simulink model "Commande_floue"  (R2016a)
settings: Solver=VariableStepAuto  StartTime=0.0  StopTime=40  RelTol=1e-3
undefined symbols (not defined in the file): A, Eg, Iscn, K, Ki, Q, Rp, Rse, T, Vocn
libraries: powerlib x14, fuzblock x1, powerlib_extras x1, simulink x1
settings Model: Creator=AIMS  LastModifiedBy=AIMS

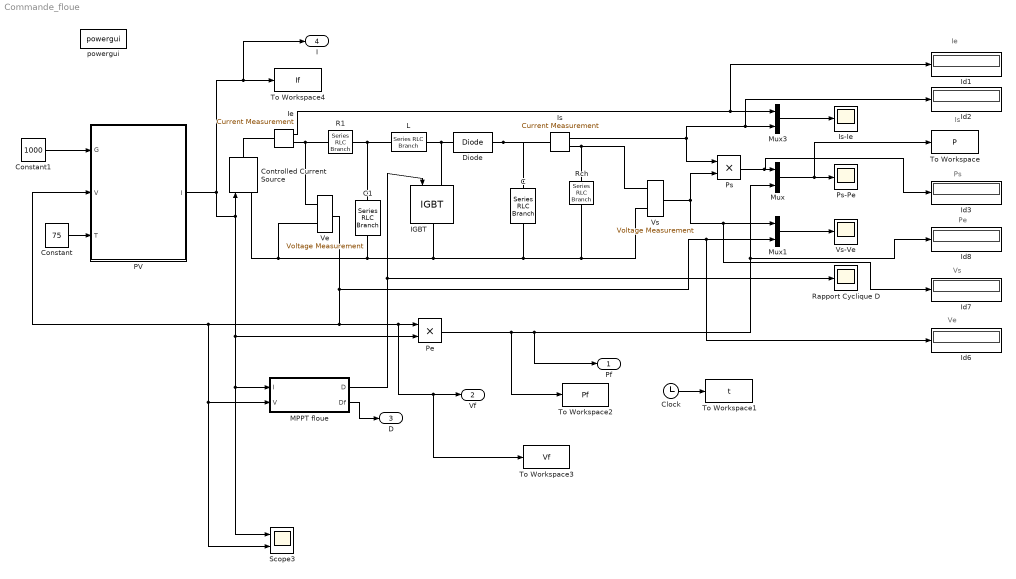
== system Commande_floue ==
  note: Ve
  note: Vs
  note: Pe
  note: Ps
  note: Is
  note: Ie
  C : powerlib/Elements/Series RLC Branch  LConnTagsString=__new0  RConnTagsString=__new0  BranchType=C  Resistance=0.01  Inductance=1.0  SetiL0=off  InitialCurrent=0  Capacitance=400e-6  Setx0=off  InitialVoltage=200  Measurements=None
  C1 : powerlib/Elements/Series RLC Branch  LConnTagsString=__new0  RConnTagsString=__new0  BranchType=C  Resistance=0.01  Inductance=1.0  SetiL0=off  InitialCurrent=0  Capacitance=2e-3  Setx0=off  InitialVoltage=0  Measurements=None
  Clock : Clock
  Constant : Constant  Value=75
  Constant1 : Constant  Value=1000
  Controlled Current Source : powerlib/Electrical Sources/Controlled Current Source  Initialize=on  Source_Type=AC  Amplitude=0  Phase=0  Frequency=0  Measurements=None
  Diode : powerlib/Power Electronics/Diode  Ron=0.001  Lon=0  Vf=0.8  IC=0  UseSnubber=off  Rs=500  Cs=250e-9  Measurements=off
  IGBT : powerlib/Power Electronics/IGBT  Ron=0.001  Lon=0  Vf=1  Tf=1e-6  Tt=2e-6  IC=0  Rs=1e5  Cs=inf  Measurements=off
  Id{1..3,6..8} (6 alike) : Display
  Ie : powerlib/Measurements/Current Measurement  Tag=PoWeRsYsTeMmEaSuReMeNt  PhasorSimulation=off  OutputType=Magnitude  PSBequivalent=0
  Is : powerlib/Measurements/Current Measurement  Tag=PoWeRsYsTeMmEaSuReMeNt  PhasorSimulation=off  OutputType=Magnitude  PSBequivalent=0
  Is-Ie : Scope
  L : powerlib/Elements/Series RLC Branch  LConnTagsString=__new0  RConnTagsString=__new0  BranchType=L  Resistance=1.0  Inductance=76.8e-6  SetiL0=off  InitialCurrent=0  Capacitance=1.0  Setx0=off  InitialVoltage=0  Measurements=None
  MPPT floue : Subsystem
  Mux : Mux  Inputs=2
  Mux1 : Mux  Inputs=2
  Mux3 : Mux  Inputs=2
  PV : Subsystem
  Pe : Product  RndMeth=Zero
  Ps : Product  RndMeth=Zero
  Ps-Pe : Scope
  R1 : powerlib/Elements/Series RLC Branch  LConnTagsString=__new0  RConnTagsString=__new0  BranchType=R  Resistance=0.01  Inductance=1.0  SetiL0=off  InitialCurrent=0  Capacitance=1.0  Setx0=off  InitialVoltage=0  Measurements=None
  Rapport Cyclique D : Scope
  Rch : powerlib/Elements/Series RLC Branch  LConnTagsString=__new0  RConnTagsString=__new0  BranchType=R  Resistance=5  Inductance=1.0  SetiL0=off  InitialCurrent=0  Capacitance=1.0  Setx0=off  InitialVoltage=0  Measurements=None
  Scope3 : Scope  NumInputPorts=2
  To Workspace : ToWorkspace  VariableName=P  SampleTime=-1
  To Workspace1 : ToWorkspace  VariableName=t  SampleTime=-1
  To Workspace2 : ToWorkspace  VariableName=Pf  SampleTime=-1
  To Workspace3 : ToWorkspace  VariableName=Vf  SampleTime=-1
  To Workspace4 : ToWorkspace  VariableName=If  SampleTime=-1
  Ve : powerlib/Measurements/Voltage Measurement  Tag=PoWeRsYsTeMmEaSuReMeNt  PhasorSimulation=off  OutputType=Magnitude  PSBequivalent=0
  Vs : powerlib/Measurements/Voltage Measurement  Tag=PoWeRsYsTeMmEaSuReMeNt  PhasorSimulation=off  OutputType=Magnitude  PSBequivalent=0
  Vs-Ve : Scope
  powergui : powerlib/powergui  SimulationMode=Continuous  SolverType=Tustin  SampleTime=50e-6  frequency=60  SPID=off  DisableSnubberDevices=off  DisableRonSwitches=off  DisableVfSwitches=off  SwTol=0  DisplayEquations=off  Interpol=off  ExternalGateDelay=off  methode=off  Ts=0  FunctionMessages=off  echomessages=off  HookPort=off  EnableUseOfTLC=off  x0status=blocks  frequencyindice=0  Pbase=100e6  ErrMax=1e-4  Iterations=50  UnitsV=kV  UnitsW=MW  buscounter=0  RestoreLinks=warning  ResistiveCurrentMeasurement=off  Frange=[0:2:500]  Ylog=off  Xlog=on  ShowGrid=off  save=off  variable=ZData  structure=mmmm  ZoomFFT=off  StartTime=0.0  cycles=1  DisplayStyle=1  fundamental=60  FreqAxis=off  MaxFrequency=1000  frequencyindicesteady=1  RmsSteady=1  display=off
  Pf : Outport
  Vf : Outport  Port=2
  D : Outport  Port=3
  "I  " : Outport  Port=4
  wires:
  Is/1 -> Id2/1, Mux3/2, Ps/1
  Vs/1 -> Id7/1, Mux1/1, Ps/2
  Pe/1 -> Id8/1, Mux/2, Pf/1, To Workspace2/1
  Ve/1 -> Id6/1, Mux1/2, PV/2(V), Scope3/2, MPPT floue/2(V), Pe/1, Vf/1, To Workspace3/1
  Mux/1 -> Ps-Pe/1, To Workspace/1
  Mux1/1 -> Vs-Ve/1
  Ie/1 -> Id1/1, Mux3/1
  Mux3/1 -> Is-Ie/1
  MPPT floue/1(D) -> Rapport Cyclique D/1, IGBT/1
  Clock/1 -> To Workspace1/1
  MPPT floue/2(Df) -> D/1
  Constant/1 -> PV/3(T)
  PV/1("I ") -> To Workspace4/1, "I  "/1, Controlled Current Source/1, Pe/2, Scope3/1, MPPT floue/1(I)
  Ps/1 -> Id3/1, Mux/1
  Constant1/1 -> PV/1("G ")
  connections:
  Vs/LConn2 -- Rch/RConn1 -- Controlled Current Source/LConn1 -- Ve/LConn2 -- C1/RConn1 -- IGBT/RConn1 -- C/RConn1
  Diode/RConn1 -- C/LConn1 -- Is/LConn1
  Diode/LConn1 -- IGBT/LConn1 -- L/RConn1
  Is/RConn1 -- Vs/LConn1 -- Rch/LConn1
  Ve/LConn1 -- Ie/RConn1 -- R1/RConn1
  R1/LConn1 -- C1/LConn1 -- L/LConn1
  Controlled Current Source/RConn1 -- Ie/LConn1

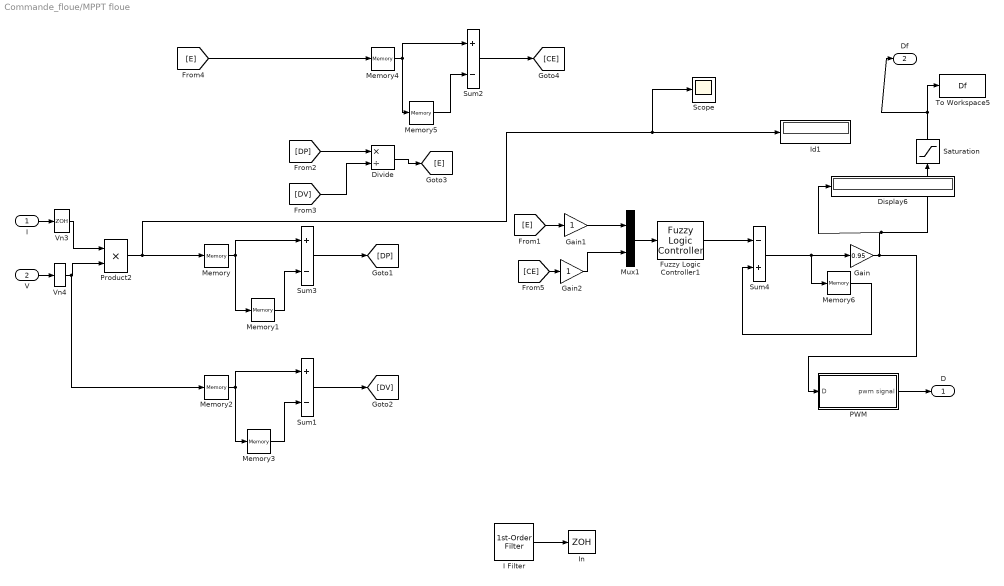
== system Commande_floue/MPPT floue ==
  I : Inport
  V : Inport  Port=2
  Display6 : Display
  Divide : Product  Inputs=*/
  Fuzzy Logic Controller1 : fuzblock/Fuzzy Logic  Controller  fis=sari
  Gain : Gain  Gain=0.95
  Gain1 : Gain
  Gain2 : Gain
  I Filter : powerlib_extras/Control  Blocks/1st-Order  Filter  FilterType=Lowpass  Tc=1e-3  Initialize=off  Vac_Init=[0.8 -25 60]  Vdc_Init=-0.4  PlotResponse=off  param1=[1 500 1]
  Id1 : Display
  In : ZeroOrderHold  SampleTime=4e-4
  Memory{,1..6} (7 alike) : Memory
  Mux1 : Mux  Inputs=2
  PWM : Subsystem
  Product2 : Product
  Saturation : Saturate  UpperLimit=1  LowerLimit=0
  Scope : Scope
  Sum1 : Sum  Inputs=|+-
  Sum2 : Sum  Inputs=|+-
  Sum3 : Sum  Inputs=|+-
  Sum4 : Sum  Inputs=-+
  To Workspace5 : ToWorkspace  VariableName=Df  SampleTime=-1
  Vn3 : ZeroOrderHold  SampleTime=0.01/2
  Vn4 : ZeroOrderHold  SampleTime=0.01/2
  D : Outport
  Df : Outport  Port=2
  wires:
  I/1 -> Vn3/1
  Product2/1 -> Scope/1, Id1/1, Memory/1
  Memory/1 -> Memory1/1, Sum3/1
  Memory1/1 -> Sum3/2
  Sum3/1 -> [DP]
  V/1 -> Vn4/1
  Memory2/1 -> Sum1/1, Memory3/1
  Memory3/1 -> Sum1/2
  Sum1/1 -> [DV]
  [DV] -> Divide/2
  [DP] -> Divide/1
  Divide/1 -> [E]
  [E] -> Memory4/1
  Memory4/1 -> Memory5/1, Sum2/1
  Memory5/1 -> Sum2/2
  Sum2/1 -> [CE]
  Mux1/1 -> Fuzzy Logic Controller1/1
  [E] -> Gain1/1
  [CE] -> Gain2/1
  Fuzzy Logic Controller1/1 -> Sum4/1
  Memory6/1 -> Sum4/2
  Sum4/1 -> Memory6/1, Gain/1
  Gain/1 -> PWM/1(D), Display6/1, Saturation/1
  Gain1/1 -> Mux1/1
  Gain2/1 -> Mux1/2
  ? -> I Filter/1
  I Filter/1 -> In/1
  PWM/1(pwm signal) -> D/1
  Vn3/1 -> Product2/1
  Vn4/1 -> Product2/2, Memory2/1
  Saturation/1 -> To Workspace5/1, Df/1

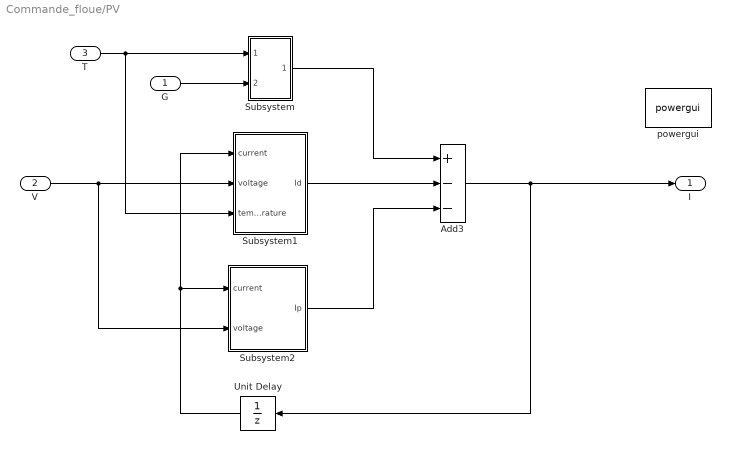
== system Commande_floue/PV ==
  "G " : Inport
  V : Inport  Port=2
  T : Inport  Port=3
  Add3 : Sum  Inputs=+--
  Subsystem : Subsystem
  Subsystem1 : Subsystem
  Subsystem2 : Subsystem
  Unit Delay : UnitDelay
  powergui : powerlib/powergui  Priority=1  SimulationMode=Continuous  SolverType=Tustin/Backward Euler (TBE)  SampleTime=50e-6  frequency=60  SPID=off  DisableSnubberDevices=off  DisableRonSwitches=off  DisableVfSwitches=off  SwTol=0  DisplayEquations=off  Interpol=off  ExternalGateDelay=off  methode=off  Ts=10  FunctionMessages=off  echomessages=off  HookPort=off  EnableUseOfTLC=off  x0status=blocks  frequencyindice=0  Pbase=100e6  ErrMax=1e-4  Iterations=50  UnitsV=kV  UnitsW=MW  buscounter=0  RestoreLinks=warning  ResistiveCurrentMeasurement=off  Frange=[0:2:500]  Ylog=off  Xlog=on  ShowGrid=off  save=off  variable=ZData  structure=0  ZoomFFT=off  StartTime=0.0  cycles=1  DisplayStyle=1  fundamental=60  FreqAxis=off  MaxFrequency=1000  frequencyindicesteady=1  RmsSteady=1  display=off
  "I " : Outport
  wires:
  Add3/1 -> "I "/1, Unit Delay/1
  "G "/1 -> Subsystem/2(In2)
  Unit Delay/1 -> Subsystem2/1("current "), Subsystem1/1(current)
  V/1 -> Subsystem2/2(voltage), Subsystem1/2(voltage)
  Subsystem1/1(Id) -> Add3/2
  Subsystem2/1(Ip) -> Add3/3
  T/1 -> Subsystem1/3(temperature), Subsystem/1(In1)
  Subsystem/1(Iph_out) -> Add3/1

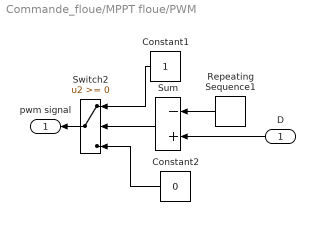
== system Commande_floue/MPPT floue/PWM ==
  D : Inport
  Constant1 : Constant  SampleTime=-1
  Constant2 : Constant  Value=0  SampleTime=-1
  Repeating Sequence1 : simulink/Sources/Repeating Sequence  rep_seq_t=[0 4e-3 4e-2]  rep_seq_y=[0 1 0]
  Sum : Sum  Inputs=-+  SaturateOnIntegerOverflow=on
  Switch2 : Switch
  pwm signal : Outport
  wires:
  Switch2/1 -> pwm signal/1
  Repeating Sequence1/1 -> Sum/1
  Sum/1 -> Switch2/2
  Constant1/1 -> Switch2/1
  Constant2/1 -> Switch2/3
  D/1 -> Sum/2

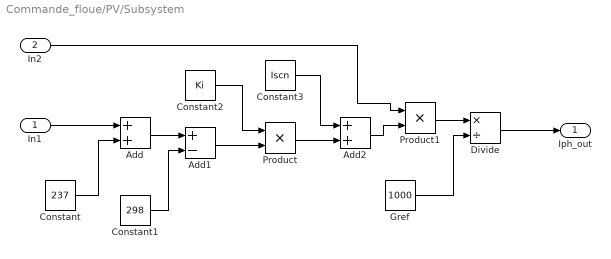
== system Commande_floue/PV/Subsystem ==
  In1 : Inport
  In2 : Inport  Port=2
  Add : Sum
  Add1 : Sum  Inputs=+-
  Add2 : Sum
  Constant : Constant  Value=237
  Constant1 : Constant  Value=298
  Constant2 : Constant  Value=Ki
  Constant3 : Constant  Value=Iscn
  Divide : Product  Inputs=*/
  "Gref " : Constant  Value=1000
  Product : Product
  Product1 : Product
  Iph_out : Outport
  wires:
  Product/1 -> Add2/2
  Divide/1 -> Iph_out/1
  In2/1 -> Product1/1
  Add2/1 -> Product1/2
  Constant1/1 -> Add1/2
  Constant3/1 -> Add2/1
  Add/1 -> Add1/1
  Constant/1 -> Add/2
  "Gref "/1 -> Divide/2
  In1/1 -> Add/1
  Add1/1 -> Product/2
  Constant2/1 -> Product/1
  Product1/1 -> Divide/1

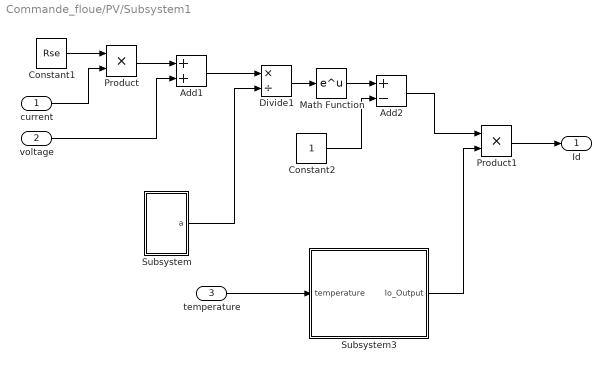
== system Commande_floue/PV/Subsystem1 ==
  current : Inport
  voltage : Inport  Port=2
  temperature : Inport  Port=3
  Add1 : Sum
  Add2 : Sum  Inputs=+-
  Constant1 : Constant  Value=Rse
  Constant2 : Constant
  Divide1 : Product  Inputs=*/
  Math Function : Math  SaturateOnIntegerOverflow=on
  Product : Product
  Product1 : Product
  Subsystem : Subsystem
  Subsystem3 : Subsystem
  Id : Outport
  wires:
  Divide1/1 -> Math Function/1
  voltage/1 -> Add1/2
  Product/1 -> Add1/1
  Constant2/1 -> Add2/2
  Product1/1 -> Id/1
  Add2/1 -> Product1/1
  Add1/1 -> Divide1/1
  Subsystem/1(a) -> Divide1/2
  Math Function/1 -> Add2/1
  current/1 -> Product/2
  Constant1/1 -> Product/1
  temperature/1 -> Subsystem3/1(temperature)
  Subsystem3/1(Io_Output) -> Product1/2

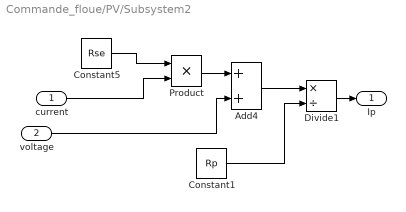
== system Commande_floue/PV/Subsystem2 ==
  "current " : Inport
  voltage : Inport  Port=2
  Add4 : Sum
  Constant1 : Constant  Value=Rp
  Constant5 : Constant  Value=Rse
  Divide1 : Product  Inputs=*/
  Product : Product
  Ip : Outport
  wires:
  "current "/1 -> Product/2
  voltage/1 -> Add4/2
  Constant5/1 -> Product/1
  Constant1/1 -> Divide1/2
  Add4/1 -> Divide1/1
  Product/1 -> Add4/1
  Divide1/1 -> Ip/1

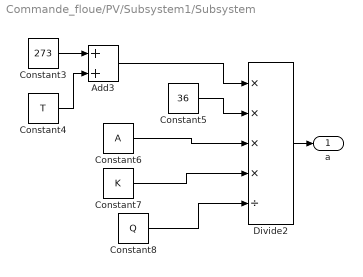
== system Commande_floue/PV/Subsystem1/Subsystem ==
  Add3 : Sum
  Constant3 : Constant  Value=273
  Constant4 : Constant  Value=T
  Constant5 : Constant  Value=36
  Constant6 : Constant  Value=A
  Constant7 : Constant  Value=K
  Constant8 : Constant  Value=Q
  Divide2 : Product  Inputs=****/
  a : Outport
  wires:
  Constant3/1 -> Add3/1
  Add3/1 -> Divide2/1
  Constant8/1 -> Divide2/5
  Divide2/1 -> a/1
  Constant5/1 -> Divide2/2
  Constant4/1 -> Add3/2
  Constant7/1 -> Divide2/4
  Constant6/1 -> Divide2/3

== system Commande_floue/PV/Subsystem1/Subsystem3 ==
  temperature : Inport
  Product2 : Product
  Subsystem1 : Subsystem
  Subsystem2 : Subsystem
  Io_Output : Outport
  wires:
  Subsystem1/1(Io1) -> Product2/2
  Subsystem2/1(Ioref) -> Product2/1
  Product2/1 -> Io_Output/1
  temperature/1 -> Subsystem1/1(Temper)

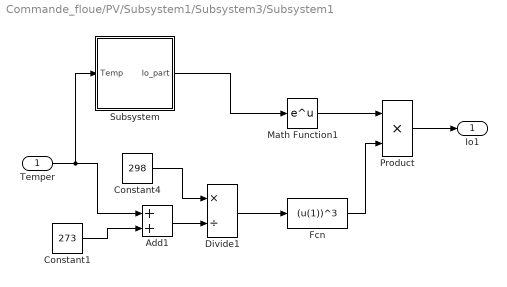
== system Commande_floue/PV/Subsystem1/Subsystem3/Subsystem1 ==
  Temper : Inport
  Add1 : Sum
  Constant1 : Constant  Value=273
  Constant4 : Constant  Value=298
  Divide1 : Product  Inputs=*/
  Fcn : Fcn  Expr=(u(1))^3
  Math Function1 : Math  SaturateOnIntegerOverflow=on
  Product : Product
  Subsystem : Subsystem
  Io1 : Outport
  wires:
  Constant1/1 -> Add1/2
  Temper/1 -> Subsystem/1(Temp), Add1/1
  Add1/1 -> Divide1/2
  Constant4/1 -> Divide1/1
  Divide1/1 -> Fcn/1
  Fcn/1 -> Product/2
  Math Function1/1 -> Product/1
  Subsystem/1(Io_part) -> Math Function1/1
  Product/1 -> Io1/1

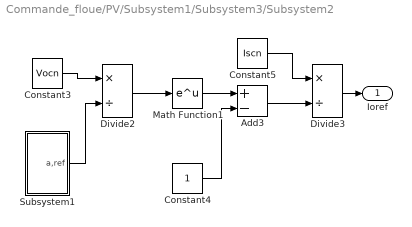
== system Commande_floue/PV/Subsystem1/Subsystem3/Subsystem2 ==
  Add3 : Sum  Inputs=+-
  Constant3 : Constant  Value=Vocn
  Constant4 : Constant
  Constant5 : Constant  Value=Iscn
  Divide2 : Product  Inputs=*/
  Divide3 : Product  Inputs=*/
  Math Function1 : Math  SaturateOnIntegerOverflow=on
  Subsystem1 : Subsystem
  Ioref : Outport
  wires:
  Subsystem1/1(a,ref) -> Divide2/2
  Constant5/1 -> Divide3/1
  Constant4/1 -> Add3/2
  Divide2/1 -> Math Function1/1
  Add3/1 -> Divide3/2
  Divide3/1 -> Ioref/1
  Math Function1/1 -> Add3/1
  Constant3/1 -> Divide2/1

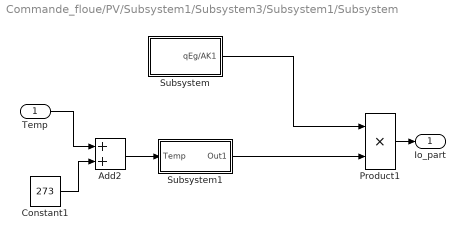
== system Commande_floue/PV/Subsystem1/Subsystem3/Subsystem1/Subsystem ==
  Temp : Inport
  Add2 : Sum
  Constant1 : Constant  Value=273
  Product1 : Product
  Subsystem : Subsystem
  Subsystem1 : Subsystem
  Io_part : Outport
  wires:
  Product1/1 -> Io_part/1
  Constant1/1 -> Add2/2
  Temp/1 -> Add2/1
  Add2/1 -> Subsystem1/1(Temp)
  Subsystem1/1(Out1) -> Product1/2
  Subsystem/1(qEg/AK1) -> Product1/1

== system Commande_floue/PV/Subsystem1/Subsystem3/Subsystem2/Subsystem1 ==
  Constant3 : Constant  Value=298
  Constant5 : Constant  Value=36
  Constant6 : Constant  Value=A
  Constant7 : Constant  Value=K
  Constant8 : Constant  Value=Q
  Divide2 : Product  Inputs=****/
  a,ref : Outport
  wires:
  Constant3/1 -> Divide2/1
  Constant8/1 -> Divide2/5
  Divide2/1 -> a,ref/1
  Constant5/1 -> Divide2/2
  Constant7/1 -> Divide2/4
  Constant6/1 -> Divide2/3

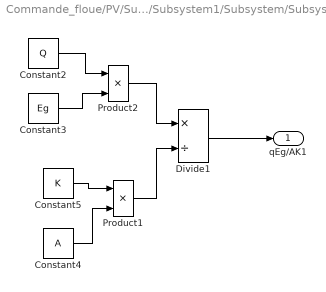
== system Commande_floue/PV/Subsystem1/Subsystem3/Subsystem1/Subsystem/Subsystem ==
  Constant2 : Constant  Value=Q
  Constant3 : Constant  Value=Eg
  Constant4 : Constant  Value=A
  Constant5 : Constant  Value=K
  Divide1 : Product  Inputs=*/
  Product1 : Product
  Product2 : Product
  qEg/AK1 : Outport
  wires:
  Constant3/1 -> Product2/2
  Constant2/1 -> Product2/1
  Constant5/1 -> Product1/1
  Constant4/1 -> Product1/2
  Product2/1 -> Divide1/1
  Product1/1 -> Divide1/2
  Divide1/1 -> qEg/AK1/1

== system Commande_floue/PV/Subsystem1/Subsystem3/Subsystem1/Subsystem/Subsystem1 ==
  Temp : Inport
  Add1 : Sum  Inputs=+-
  Constant2 : Constant  Value=1/298
  Fcn : Fcn  Expr=1/u
  Out1 : Outport
  wires:
  Constant2/1 -> Add1/1
  Temp/1 -> Fcn/1
  Add1/1 -> Out1/1
  Fcn/1 -> Add1/2
